simulink model "test"  (Simulink 7.6)
settings: Solver=ode3  StartTime=0.0  StopTime=inf  FixedStep=0.05  RelTol=1e-3
libraries: aerolibanimutils x1
settings Model: Creator=Owen  LastModifiedBy=Owen

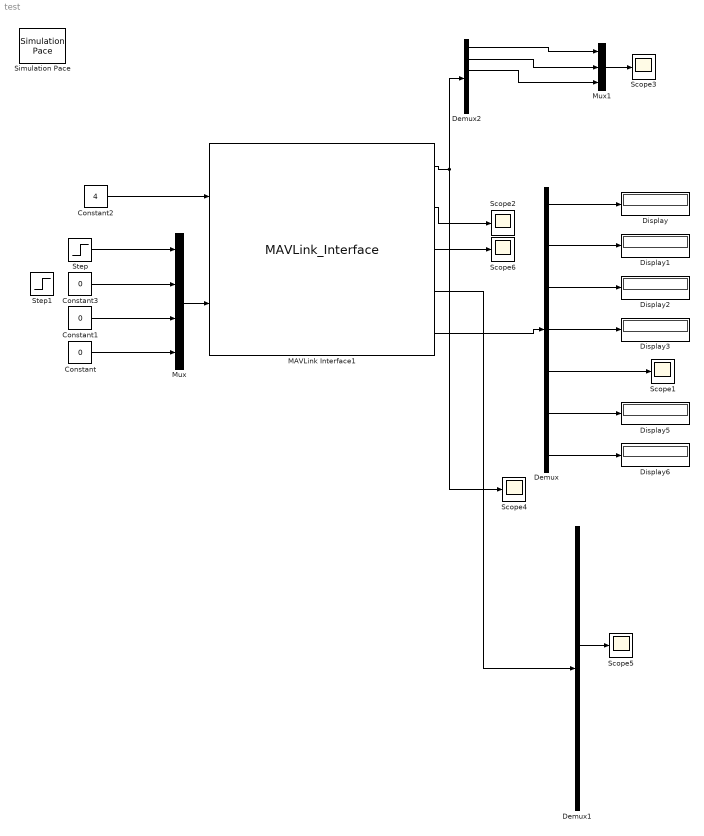
== system test ==
  Constant : Constant  Value=0
  Constant1 : Constant  Value=0
  Constant2 : Constant  Value=4
  Constant3 : Constant  Value=0
  Demux : Demux  Outputs=7
  Demux1 : Demux  Outputs=6
  Demux2 : Demux  Outputs=6
  Display{,1..3,5..6} (6 alike) : Display
  MAVLink Interface1 : S-Function  FunctionName=MAVLink_Interface  Parameters=COM_Port,Baud_Rate,IP_ADDRESS,IP_PORT,SYS_ID,COMP_ID,COMP_TARG,MSG_INPUT,MSG_OUTPUT  EnableBusSupport=off  mask{COM_Port='', Baud_Rate=115200, IP_ADDRESS='131.231.124.183', IP_PORT=5013, SYS_ID=255, COMP_ID=0, COMP_TARG='/aircraft/LU-WOTA/APM', HEART_BEAT=off, ATTITUDE_OUT=on, RAW_IMU=off, POSITION_OUT=on, POSITION_OUT2=on, VFR_HUD=on, RC_SCALED=off, SERVO_OUT_RAW=off, SYS_STATUS=on, SET_MODE=on, DATA_STREAM=off, ATTITUDE_COMMAND=on, RC_OVERRIDE=off, ATTITUDE_IN=off, GPS_RAW_IN=off, VFR_HUD_IN=off}
      mask prompts: COM_Port "COM Port"; Baud_Rate "Baud Rate"; IP_ADDRESS "IP Address"; IP_PORT "Port"; SYS_ID "System ID"; COMP_ID "Component ID"; COMP_TARG "Target Component"; HEART_BEAT "Heartbeat"; ATTITUDE_OUT "Attitude"; RAW_IMU "Raw IMU"; POSITION_OUT "Global Position"; POSITION_OUT2 "Global Position 2"; VFR_HUD "VFR HUD"; RC_SCALED "Scaled RC Channels"; SERVO_OUT_RAW "Raw Servo Positions"; SYS_STATUS "System Status"; SET_MODE "Mode"; DATA_STREAM "Datastream Request"; ATTITUDE_COMMAND "Attitude Command"; RC_OVERRIDE "RC Override"; ATTITUDE_IN "Attitude (HIL)"; GPS_RAW_IN "Raw GPS (HIL)"; VFR_HUD_IN "VFR HUD (HIL)"
      mask init:
      | MSG_ID_NUM_INPUT = [uint8(11) uint8(66) uint8(70) uint8(55) uint8(30) uint8(32) uint8(73)];
      | MSG_ID_NAME_INPUT = [SET_MODE DATA_STREAM RC_OVERRIDE ATTITUDE_COMMAND ATTITUDE_IN GPS_RAW_IN VFR_HUD_IN];
      | 
      | MSG_ID_NUM_OUTPUT = [uint8(0) uint8(30) uint8(28) uint8(73) uint8(32) uint8(74) uint8(36) uint8(37) uint8(34)];
      | MSG_ID_NAME_OUTPUT = [HEART_BEAT ATTITUDE_OUT RAW_IMU VFR_HUD POSITION_OUT2 POSITION_OUT RC_SCALED SERVO_OUT_RAW SYS_STATUS];
      | 
      | idx_input = find(MSG_ID_NAME_INPUT);
      | MSG_INPUT = MSG_ID_NUM_INPUT(idx_input);
      | 
      | idx_output = find(MSG_ID_NAME_OUTPUT);
      | MSG_OUTPUT = MSG_ID_NUM_OUTPUT(idx_output);
      mask TabNameString: Connection,Connection,Connection,Connection,MAVLink,MAVLink,MAVLink,Outputs,Outputs,Outputs,Outputs,Outputs,Outputs,Outputs,Outputs,Outputs,Inputs,Inputs,Inputs,Inputs,Inputs,Inputs,Inputs
      mask Display:
      | %Label block
      | 
      | if (~strcmp(COM_Port, ''))
      | fprintf('MAVLink Serial\n%s\n%dbps', COM_Port,  Baud_Rate)
      | end
      | if (~strcmp(IP_ADDRESS, ''))
      | fprintf('MAVLink TCP\n%s:%d', IP_ADDRESS,  IP_PORT)
      | end
      | fprintf('\n\n\n\n\n%d:%d\n%s', SYS_ID, COMP_ID, COMP_TARG)
      | 
      | 
      | %Label input ports
      | 
      | in = 1;
      | if (SET_MODE == 1)
      |     port_label('input', in, 'Mode');
      |     in = in + 1;
      | end
      | if (DATA_STREAM == 1)
      |     port_label('input', in, 'Datastream Request');
      |     in = in + 1;
      | end
      | if (ATTITUDE_COMMAND == 1)
      |     port_label('input', in, 'Attitude Command');
      |     in = in + 1;
      | end
      | if (ATTITUDE_IN == 1)
      |     port_label('input', in, 'Attitude (HIL)');
      |     in = in + 1;
      | end
      | if (GPS_RAW_IN == 1)
      |     port_label('input', in, 'Raw GPS (HIL)');
      |     in = in + 1;
      | end
      | if (VFR_HUD_IN == 1)
      |     port_label('input', in, 'VFR HUD (HIL)');
      |     in = in + 1;
      | end
      | 
      | %Label output ports
      | 
      | out = 1;
      | if (HEART_BEAT == 1)
      |     port_label('output', out, 'Heartbeat');
      |     out = out + 1;
      | end
      | if (ATTITUDE_OUT == 1)
      |     port_label('output', out, 'Attitude');
      |     out = out + 1;
      | end
      | if (RAW_IMU == 1)
      |     port_label('output', out, 'Raw IMU');
      |     out = out + 1;
      | end
      | if (POSITION_OUT == 1)
      |     port_label('output', out, 'Global Position');
      |     out = out + 1;
      | end
      | if (POSITION_OUT2 == 1)
      |     port_label('output', out, 'Global Position 2');
      |     out = out + 1;
      | end
      | if (VFR_HUD == 1)
      |     port_label('output', out, 'VFR HUD');
      |     out = out + 1;
      | end
      | if (RC_SCALED == 1)
      |     port_label('output', out, 'Scaled RC Channels');
      |     out = out + 1;
      | end
      | if (SERVO_OUT_RAW == 1)
      |     port_label('output', out, 'Raw Servo Output');
      |     out = out + 1;
      | end
      | if (SYS_STATUS == 1)
      |     port_label('output', out, 'System Status');
      |     out = out + 1;
      | end
  Mux : Mux
  Mux1 : Mux  Inputs=3
  Scope{1..6} (6 alike) : Scope
      Scope1 settings: TimeRange=7  YMin=0  YMax=13000
      Scope2 settings: TimeRange=7  YMax=100  SaveName=ScopeData2
      Scope3 settings: TimeRange=7  YMin=-1.2  YMax=0.1  SaveName=ScopeData3
      Scope4 settings: TimeRange=7  YMin=-1  YMax=1
      Scope5 settings: TimeRange=7  YMin=115.9  YMax=128.1  SaveName=ScopeData4
      Scope6 settings: TimeRange=7  YMax=105  SaveName=ScopeData5
  Simulation Pace : aerolibanimutils/Simulation Pace  SimulationPace=1  SleepMode=MATLAB Thread  OutputPaceError=off  SampleTime=1/10
      settings: AttributesFormatString=%<SimulationPace> sec/sec
  Step : Step  Time=15  Before=-1  SampleTime=0
  Step1 : Step  Time=15  Before=0.2  SampleTime=0
  wires:
  Demux/2 -> Display1/1
  Demux/3 -> Display2/1
  Demux/4 -> Display3/1
  Demux/5 -> Scope1/1
  Demux/6 -> Display5/1
  Demux/7 -> Display6/1
  Constant/1 -> Mux/4
  Constant1/1 -> Mux/3
  Step/1 -> Mux/1
  Mux1/1 -> Scope3/1
  Demux/1 -> Display/1
  MAVLink Interface1/1 -> Scope4/1, Demux2/1
  MAVLink Interface1/2 -> Scope2/1
  MAVLink Interface1/3 -> Scope6/1
  MAVLink Interface1/5 -> Demux/1
  MAVLink Interface1/4 -> Demux1/1
  Demux1/3 -> Scope5/1
  Demux2/1 -> Mux1/1
  Demux2/2 -> Mux1/2
  Demux2/3 -> Mux1/3
  Mux/1 -> MAVLink Interface1/2
  Constant2/1 -> MAVLink Interface1/1
  Constant3/1 -> Mux/2
